simulink model "simulator_linearbicycle"  (R2025b)
settings: Solver=ode45  StartTime=0.0  StopTime=20  FixedStep=1e-4  RelTol=1e-3
undefined symbols (not defined in the file): v0, x0
settings Model: Creator=ateveraz  LastModifiedBy=ateveraz

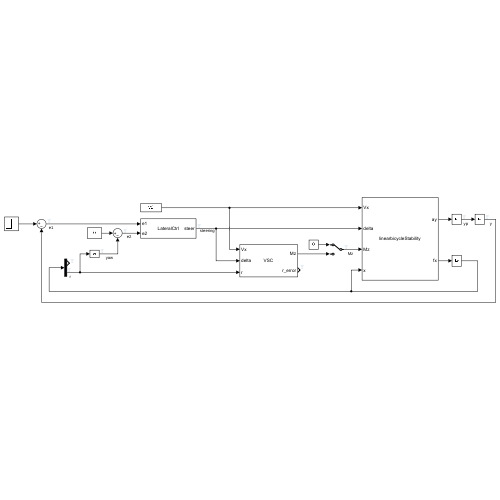
[thumbnail: Simulink's stored preview of the top-level diagram]
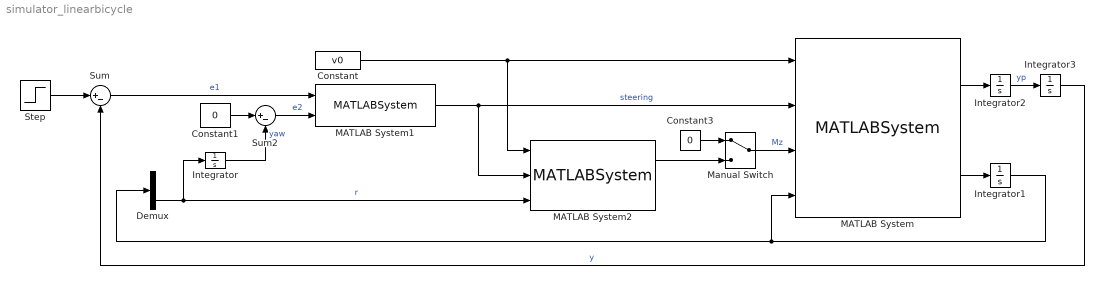
== system simulator_linearbicycle ==
  Constant : Constant  Value=v0
  Constant1 : Constant  Value=0
  Constant3 : Constant  Value=0
  Demux : Demux  Outputs=2
  Integrator : Integrator
  Integrator1 : Integrator  InitialCondition=x0
  Integrator2 : Integrator
  Integrator3 : Integrator
  MATLAB System : MATLABSystem  System=linearbicycleStability  SimulateUsing=Interpreted execution
      mask Type: linearbicycleStability
  MATLAB System1 : MATLABSystem  System=LateralCtrl  Kp=1  Kd=2  SimulateUsing=Interpreted execution
      mask Type: LateralCtrl
  MATLAB System2 : MATLABSystem  System=VSC  Kp=10  Kd=0  SimulateUsing=Interpreted execution
      mask Type: VSC
  Manual Switch : ManualSwitch
  Step : Step  Time=5  Before=5  After=20  SampleTime=0
  Sum : Sum  Inputs=|+-
  Sum2 : Sum  Inputs=|+-
  wires:
  Integrator1/1 -> MATLAB System/4, Demux/1
  Constant/1 -> MATLAB System2/1, MATLAB System/1
  Integrator2/1 -> Integrator3/1  "yp"
  Integrator3/1 -> Sum/2  "y"
  MATLAB System1/1 -> MATLAB System/2, MATLAB System2/2  "steering"
  Sum/1 -> MATLAB System1/1  "e1"
  MATLAB System2/1 -> Manual Switch/2
  Constant1/1 -> Sum2/1
  Demux/2 -> Integrator/1, MATLAB System2/3  "r"
  MATLAB System/1 -> Integrator2/1
  MATLAB System/2 -> Integrator1/1
  Manual Switch/1 -> MATLAB System/3  "Mz"
  Constant3/1 -> Manual Switch/1
  Step/1 -> Sum/1
  Sum2/1 -> MATLAB System1/2  "e2"
  Integrator/1 -> Sum2/2  "yaw"
